simulink model "Acquisition"  (R2017a)
settings: Solver=VariableStepAuto  StartTime=0.0  StopTime=1  RelTol=1e-3
undefined symbols (not defined in the file): Radix
libraries: dspxfrm3 x3, dspswit3 x2, dspbuff3 x1, simulink_extras x1
settings Model: Creator=Alam  LastModifiedBy=Alam
settings SolverCC: AutoInsertRateTranBlk=on
settings DataIOCC: LimitDataPoints=on  SaveOutput=off  SignalLogging=off  SaveTime=off
settings OptimizationCC: LifeSpan=inf
settings DebuggingCC: AlgebraicLoopMsg=none  SingleTaskRateTransMsg=error  AllowSymbolicDim=off  SFUnexpectedBacktrackingDiag=warning  SFNoUnconditionalDefaultTransitionDiag=warning  SFExecutionAtInitializationDiag=none
settings GRTTargetCC: TargetLangStandard=C89/C90 (ANSI)  GeneratePreprocessorConditionals=Disable all

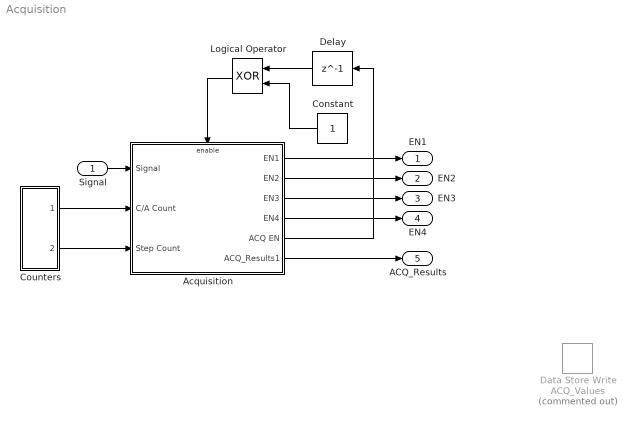
== system Acquisition ==
  Signal : Inport
  Acquisition : Subsystem
  Constant : Constant
  Counters : Subsystem  TreatAsAtomicUnit=on
  Data Store Write : DataStoreWrite  Commented=on  DataStoreName=ACQ_Values
  Delay : Delay  DelayLength=1  InitialCondition=0
  Logical Operator : Logic  Operator=XOR  AllPortsSameDT=off  OutDataTypeStr=boolean
  EN1 : Outport
  EN2 : Outport  Port=2
  EN3 : Outport  Port=3
  EN4 : Outport  Port=4
  ACQ_Results : Outport  Port=5
  wires:
  Signal/1 -> Acquisition/1(Signal)
  Delay/1 -> Logical Operator/1
  Constant/1 -> Logical Operator/2
  Counters/1(Out1) -> Acquisition/2(C/A Count)
  Counters/2(Out2) -> Acquisition/3(Step Count)
  Acquisition/1(EN1) -> EN1/1
  Acquisition/2(EN2) -> EN2/1
  Acquisition/3(EN3) -> EN3/1
  Acquisition/4(EN4) -> EN4/1
  Logical Operator/1 -> Acquisition/Enable
  Acquisition/5(ACQ EN) -> Delay/1
  Acquisition/6(ACQ_Results1) -> ACQ_Results/1

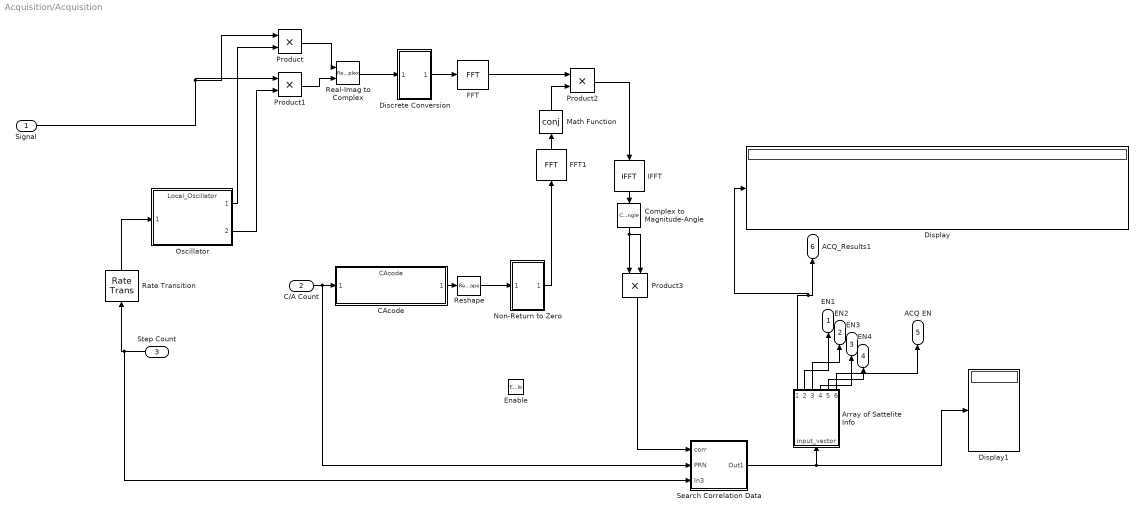
== system Acquisition/Acquisition ==
  Signal : Inport
  C/A Count : Inport  Port=2
  Step Count : Inport  Port=3
  Enable : EnablePort
  Array of Sattelite Info : MATLAB Function  TreatAsAtomicUnit=on  SystemSampleTime=0.001
  CAcode : ModelReference  ModelNameDialog=CAcode.mdl  SimulationMode=Normal  ModelReferenceVersion=1.53
  Complex to Magnitude-Angle : ComplexToMagnitudeAngle  Output=Magnitude
  "Discrete Conversion " : Subsystem  TreatAsAtomicUnit=on
  Display : Display
  Display1 : Display
  FFT : dspxfrm3/FFT  FFTImplementation=Radix-2  CompMethod=Table lookup  TableOpt=NEW  TableOptActive=Speed  BitRevOrder=off  Normalize=off  InheritFFTLength=on  FFTLength=64  WrapInput=on  roundingMode=Floor  overflowMode=off  firstCoeffDataTypeStr=Inherit: Same word length as input  firstCoeffLastDataTypeStr=Inherit: Same word length as input  outputMin=[]  outputMax=[]
  FFT1 : dspxfrm3/FFT  FFTImplementation=Radix-2  CompMethod=Table lookup  TableOpt=NEW  TableOptActive=Speed  BitRevOrder=off  Normalize=off  InheritFFTLength=on  FFTLength=64  WrapInput=on  roundingMode=Floor  overflowMode=off  firstCoeffDataTypeStr=Inherit: Same word length as input  firstCoeffLastDataTypeStr=Inherit: Same word length as input  outputMin=[]  outputMax=[]
  IFFT : dspxfrm3/IFFT  FFTImplementation=Radix-2  CompMethod=Table lookup  TableOpt=NEW  TableOptActive=Speed  BitRevOrder=off  cs_in=off  Normalize=on  InheritFFTLength=on  FFTLength=64  WrapInput=on  mode=Complex  outSamplingMode=Sample based  roundingMode=Floor  overflowMode=off  firstCoeffDataTypeStr=Inherit: Same word length as input  firstCoeffLastDataTypeStr=Inherit: Same word length as input  outputMin=[]  outputMax=[]
      settings: SourceProductName=DSP System Toolbox
  Math Function : Math  Operator=conj  SaturateOnIntegerOverflow=on
  Non-Return to Zero : Subsystem  TreatAsAtomicUnit=on
  Oscillator : ModelReference  ModelNameDialog=Local_Oscillator.slx  SimulationMode=Normal  ModelReferenceVersion=1.41
  Product{,1..3} (4 alike) : Product
  Rate Transition : RateTransition
  Real-Imag to Complex : RealImagToComplex
  Reshape : Reshape  OutputDimensionality=Column vector (2-D)
  Search Correlation Data : Subsystem  TreatAsAtomicUnit=on
  EN1 : Outport  SampleTime=0.021
  EN2 : Outport  Port=2  SampleTime=0.021
  EN3 : Outport  Port=3  SampleTime=0.021
  EN4 : Outport  Port=4  SampleTime=0.021
  ACQ EN : Outport  Port=5  SampleTime=0.021
  ACQ_Results1 : Outport  Port=6  SampleTime=0.021
  wires:
  FFT1/1 -> Math Function/1
  CAcode/1 -> Reshape/1
  Product1/1 -> Real-Imag to Complex/2
  IFFT/1 -> Complex to Magnitude-Angle/1
  Rate Transition/1 -> Oscillator/1
  Oscillator/1 -> Product/2
  Math Function/1 -> Product2/2
  Complex to Magnitude-Angle/1 -> Product3/1, Product3/2
  Step Count/1 -> Search Correlation Data/3(In3), Rate Transition/1
  "Discrete Conversion "/1(Out1) -> FFT/1
  FFT/1 -> Product2/1
  Reshape/1 -> Non-Return to Zero/1(In1)
  Real-Imag to Complex/1 -> "Discrete Conversion "/1(In1)
  Non-Return to Zero/1(Out1) -> FFT1/1
  C/A Count/1 -> Search Correlation Data/2(PRN), CAcode/1
  Product2/1 -> IFFT/1
  Product/1 -> Real-Imag to Complex/1
  Oscillator/2 -> Product1/2
  Signal/1 -> Product/1, Product1/1
  Product3/1 -> Search Correlation Data/1(corr)
  Array of Sattelite Info/3(EN2) -> EN2/1
  Array of Sattelite Info/5(EN4) -> EN4/1
  Array of Sattelite Info/6(ACQ_EN) -> ACQ EN/1
  Array of Sattelite Info/1(Visible_Satellites) -> ACQ_Results1/1, Display/1
  Search Correlation Data/1(Out1) -> Array of Sattelite Info/1(input_vector), Display1/1
  Array of Sattelite Info/4(EN3) -> EN3/1
  Array of Sattelite Info/2(EN1) -> EN1/1

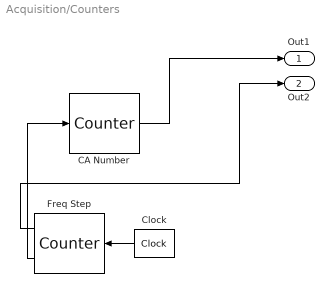
== system Acquisition/Counters ==
  CA Number : dspswit3/Counter  Direction=Up  CountEvent=Rising edge  CounterSize=User defined  MaxCount=31  InitialCount=0  Output=Count  HitValue=32  ResetInput=off  SamplesPerFrame=1  Ts=1  CntDtype=double  HitDtype=Logical
  Clock : simulink_extras/Flip Flops/Clock  period=0.001
  Freq Step : dspswit3/Counter  Direction=Up  CountEvent=Rising edge  CounterSize=User defined  MaxCount=20  InitialCount=0  Output=Count and Hit  HitValue=0  ResetInput=off  SamplesPerFrame=1  Ts=1  CntDtype=double  HitDtype=Logical
  Out1 : Outport
  Out2 : Outport  Port=2
  wires:
  Clock/1 -> Freq Step/1
  Freq Step/2 -> CA Number/1
  CA Number/1 -> Out1/1
  Freq Step/1 -> Out2/1

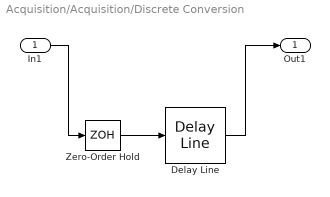
== system Acquisition/Acquisition/Discrete Conversion  ==
  In1 : Inport
  Delay Line : dspbuff3/Delay Line  siz=32768  ic=0  directfeed=off  enable_output=off  hold_output=off  OutputFrames=off
      settings: SourceProductName=DSP System Toolbox  SourceProductBaseCode=DS
  Zero-Order Hold : ZeroOrderHold  SampleTime=3.05175781e-8
  Out1 : Outport  SampleTime=0.001
  wires:
  Delay Line/1 -> Out1/1
  Zero-Order Hold/1 -> Delay Line/1
  In1/1 -> Zero-Order Hold/1

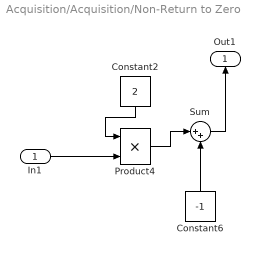
== system Acquisition/Acquisition/Non-Return to Zero ==
  In1 : Inport
  Constant2 : Constant  Value=2
  Constant6 : Constant  Value=-1
  Product4 : Product
  Sum : Sum  Inputs=|++
  Out1 : Outport
  wires:
  Sum/1 -> Out1/1
  Constant2/1 -> Product4/1
  Product4/1 -> Sum/1
  In1/1 -> Product4/2
  Constant6/1 -> Sum/2

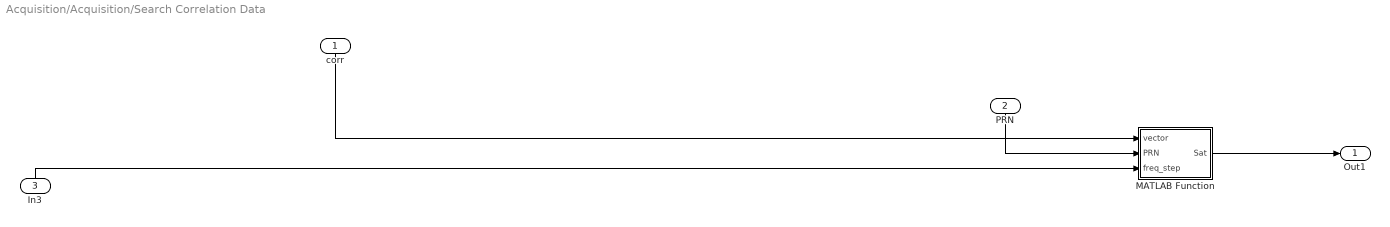
== system Acquisition/Acquisition/Search Correlation Data ==
  corr : Inport  PortDimensions=[32768 1]  SampleTime=0.001
  PRN : Inport  Port=2  SampleTime=0.001
  In3 : Inport  Port=3  SampleTime=0.001
  MATLAB Function : MATLAB Function  TreatAsAtomicUnit=on  SystemSampleTime=0.001
  Out1 : Outport
  wires:
  MATLAB Function/1(Sat) -> Out1/1
  In3/1 -> MATLAB Function/3(freq_step)
  corr/1 -> MATLAB Function/1(vector)
  PRN/1 -> MATLAB Function/2(PRN)

== matlab function Acquisition/Array of Sattelite Info ==
  data: input_vector input; Visible_Satellites output; EN1 output; EN2 output; EN3 output; EN4 output; ACQ_EN output
function [Visible_Satellites, EN1, EN2, EN3, EN4, ACQ_EN]= sort_store(input_vector)
persistent output_vector;
persistent found;
persistent find1;
persistent find2;
persistent find3;
persistent find4;
persistent PRN_prev;
persistent flag;
persistent ACQ_off;
threshold = 2*10^7;
if isempty(find4)
    find1=0;
    find2=0;
    find3=0;
    find4=0;
    flag=0;
    PRN_prev=0;
    ACQ_off=0;
end
if isempty(found)
    found=0;
end
if isempty(output_vector)
    output_vector=zeros(6,4);
end

if input_vector(1,1)>threshold
    for x = 1:6
        if (output_vector(x,1)== 0) || (output_vector(x,2)==input_vector(2,1))
    output_vector(x,1)=input_vector(1,1); %Correlation Value
    output_vector(x,2)=input_vector(2,1); %PRN
    output_vector(x,3)=input_vector(3,1); %Frequency
    output_vector(x,4)=input_vector(4,1); %Code Phase
    flag=1;
        break
        end
    end
end

if(PRN_prev~=input_vector(2,1))&& (flag==1)
    flag=0;
    found=found+1;
end
PRN_prev=input_vector(2,1);
if (found>=1)
    find1=1;
end
if (found>=2)
    find2=1;
end
if (found>=3)
    find3=1;
end
if (found>=4)
    find4=1;
    ACQ_off=1;
end
Visible_Satellites = output_vector;
EN1=find1;
EN2=find2;
EN3=find3;
EN4=find4;
ACQ_EN=ACQ_off;

== matlab function Acquisition/Search Correlation Data/MATLAB Function ==
  data: vector input; Sat output; PRN input; freq_step input
function Sat = find(vector, PRN, freq_step)
PRN=PRN+1;
freq_step=freq_step-2;
Freq =9207000+freq_step*500-5000;
persistent PRN_prev;
if isempty(PRN_prev)
    PRN_prev=0;
end
persistent sat_vector;
if isempty(sat_vector)
    sat_vector=zeros(5,1);
end
if PRN_prev ~= PRN
    sat_vector(1,1)=0;
    sat_vector(2,1)=0;
    sat_vector(3,1)=0;
    sat_vector(4,1)=0;
    sat_vector(5,1)=0;
end
for x = 1:32768
    if (vector(x,1) >= sat_vector(1,1))
       sat_vector(1,1)=vector(x,1);
       sat_vector(2,1)=PRN;
       sat_vector(3,1)=Freq;    
       sat_vector(4,1)=floor((x-1)/32);
       sat_vector(5,1)=(freq_step);
    end
end 
PRN_prev=PRN;
Sat = sat_vector;
